simulink model "eVTOL_PX4_2023b"  (R2024b)
settings: Solver=ode4  StartTime=0  StopTime=inf  FixedStep=0.01  RelTol=1e-3
values from neighbouring files (symbols this model uses):
  aDl =     [initdata.mat]
  aDr =     [initdata.mat]
  aDyn =     [initdata.mat]
  Airport = init_airport('PHNL')    [initdata_HIL_eVTOL.m]
  aLat =     [initdata.mat]
  aLon =     [initdata.mat]
  D = Prop.D    [EOM_dt_MC.m]    (also in EOM_get_alf_dt_de_prop_evtol.m = CD * QS)
  dt0 = X(2)    [EOM_get_alf_dt_de_prop_evtol.m]    (also in initdata.mat = 0.258252593971; initdata_HIL_eVTOL.m = EOM_dt_MC)
  EAS0 = TAS0 / EAS2TAS    [initdata_HIL_eVTOL.m]
  FCS = init_FCS    [initdata_HIL_eVTOL.m]
  General = init_layoutdata    [EOM_dt_MC.m]    (also in build_optimized_CA.m; initdata.mat = ; initdata_HIL_eVTOL.m)
  h0 = Con(1)    [EOM_get_alf_dt_de_prop_evtol.m]    (also in initdata.mat = 450; initdata_HIL_eVTOL.m = 50)
  mass = Con(3)    [EOM_get_alf_dt_de_prop_evtol.m]    (also in initdata.mat = 2255.54; initdata_HIL_eVTOL.m = 7)
  Motor = init_motor_evtol    [EOM_dt_MC.m]    (also in initdata.mat = []; initdata_HIL_eVTOL.m)
  Prop = init_propeller_evtol_new    [EOM_dt_MC.m]    (also in initdata_HIL_eVTOL.m)
  R2D = 180/pi    (= 57.2957795131)    [EOM_get_alf_dt_de_prop_evtol.m]    (also in init_FCS.m; init_aerodata_evtol.m; init_airport.m; initdata.mat)
  SAMPLE_TIME = 0.01    [initdata_HIL_eVTOL.m]
  theta0 = -0.0510981441662    [initdata.mat]
undefined symbols (not defined in the file or in its folder): A1, aDa, aDe, aero, asbhl20env, B1, C1, de0, Earth, Environment, INIT_Data, InitData, Kd, Kp, magnitude, Newton, pProp, Raphson, Tc, WGS84
libraries: simulink_extras x63, vrlib x48, sharedtransform x28, simulink x22, slpidlib x20, sharedutil x20, matrix_library x18, aerolibwindfilters x12, aerolibobsolete x8, aerolibasang x8, aerolibatmos2 x6, aerolibfltsims x6
(part 14 of 17)

== system eVTOL_PX4_2023b/Subsystem2/airframe/force moment/aero F&M in body axis/Aerodynamic Coefficients ==
  Incid : Inport
  mach : Inport  Port=2
  pqrn : Inport  Port=3
  alphaDot_n : Inport  Port=4
  Act_surface : Inport  Port=5
  Actuator Increments : Subsystem  AncestorBlock=|
      | asbhl20vehicle/Vehicle/Aerodynamic/Aerodynamic
      | Coefficients/Actuator
      | Increments
      settings: LibrarySourceBlock=|
      | asbhl20vehicle/Vehicle/Aerodynamic/Aerodynamic
      | Coefficients/Actuator
      | Increments
  Basic Coefficients : Subsystem  AncestorBlock=asbhl20vehicle/Vehicle/Aerodynamic/Aerodynamic Coefficients/Datum Coefficients
      settings: LibrarySourceBlock=|
      | asbhl20vehicle/Vehicle/Aerodynamic/Aerodynamic
      | Coefficients/Datum Coefficients
  Body Rate Damping : Subsystem  AncestorBlock=|
      | asbhl20vehicle/Vehicle/Aerodynamic/Aerodynamic
      | Coefficients/Body Rate
      | Damping
      settings: LibrarySourceBlock=|
      | asbhl20vehicle/Vehicle/Aerodynamic/Aerodynamic
      | Coefficients/Body Rate
      | Damping
  CLCDCY-CXCYCZ : Subsystem
  Divide : Product  Inputs=*/
  K : Scope
  Mux1 : Mux  Inputs=2
  Scope{1..5} (5 alike) : Scope
  Selector : Selector  InputPortWidth=6  IndexOptions=Index vector (dialog)  Indices=[1 2 3]  OutputSizes=1
  Selector1 : Selector  InputPortWidth=6  IndexOptions=Index vector (dialog)  Indices=[4 5 6]  OutputSizes=1
  Selector2 : Selector  InputPortWidth=3  IndexOptions=Index vector (dialog)  Indices=1  OutputSizes=1
  Selector3 : Selector  InputPortWidth=3  IndexOptions=Index vector (dialog)  Indices=2  OutputSizes=1
  Sum : Sum  Inputs=3  InputSameDT=on  SaturateOnIntegerOverflow=on  OutDataTypeStr=Inherit: Same as first input
  Coeff : Outport  InitialOutput=0  VectorParamsAs1DForOutWhenUnconnected=off
  wires:
  CLCDCY-CXCYCZ/1(Cl_XYZ) -> Scope1/1, Mux1/1
  Selector1/1 -> Mux1/2, Scope5/1
  Basic Coefficients/1(cl) -> Sum/1, Scope2/1
  Selector2/1 -> Divide/1  "CL"
  Body Rate Damping/1(cl) -> Sum/3, Scope4/1
  alphaDot_n/1 -> Body Rate Damping/3(alphaDot_n)
  Mux1/1 -> Coeff/1
  pqrn/1 -> Body Rate Damping/2(pqrn)
  Actuator Increments/1(cl) -> Sum/2, Scope3/1
  Selector/1 -> Selector3/1, Selector2/1, CLCDCY-CXCYCZ/2(Cl_LDY)
  Selector3/1 -> Divide/2  "CD"
  Sum/1 -> Selector/1, Selector1/1
  Divide/1 -> K/1
  Incid/1 -> Actuator Increments/2(incid), CLCDCY-CXCYCZ/1(Incid), Body Rate Damping/1(Incid), Basic Coefficients/1(Incid)
  Act_surface/1 -> Actuator Increments/1(Actuators)
  mach/1 -> Basic Coefficients/2(mach)

== system eVTOL_PX4_2023b/Subsystem2/airframe/force moment/aero F&M in body axis/nonunit value ==
  V : Inport
  pqr : Inport  Port=2
  alphaDot : Inport  Port=3
  CA : Constant  Value=General.MAC
  Demux2 : Demux  Outputs=3
      settings: DisplayOption=none
  Gain : Gain  Gain=2  SaturateOnIntegerOverflow=on  OutDataTypeStr=Inherit: Same as input  ParamDataTypeStr=Inherit: Same as input
  Mux18 : Mux  Inputs=3
  Product{1..4} (4 alike) : Product  Inputs=/**  SaturateOnIntegerOverflow=on  OutDataTypeStr=Inherit: Same as first input
  b : Constant  Value=General.b
  pqr_n : Outport  VectorParamsAs1DForOutWhenUnconnected=off
  alphaDot_n : Outport  Port=2  VectorParamsAs1DForOutWhenUnconnected=off
  wires:
  pqr/1 -> Demux2/1
  V/1 -> Gain/1
  Product4/1 -> Mux18/2
  Product2/1 -> Mux18/3
  Gain/1 -> Product1/1, Product2/1, Product3/1, Product4/1
  b/1 -> Product1/2, Product2/2
  Demux2/3 -> Product2/3  "r"
  Demux2/2 -> Product4/3  "q"
  Demux2/1 -> Product1/3  "p"
  CA/1 -> Product4/2, Product3/2
  Mux18/1 -> pqr_n/1
  Product1/1 -> Mux18/1
  alphaDot/1 -> Product3/3
  Product3/1 -> alphaDot_n/1

== system eVTOL_PX4_2023b/UAV/airframe/Flight Conditions/Incidence, Sideslip, & Airspeed/Subsystem ==
  V : Inport
  Demux1 : Demux  Outputs=3
      settings: DisplayOption=none
  Terminator : Terminator
  w : Outport  VectorParamsAs1DForOutWhenUnconnected=off
  U : Outport  Port=2  VectorParamsAs1DForOutWhenUnconnected=off
  wires:
  Demux1/3 -> w/1
  Demux1/2 -> Terminator/1
  V/1 -> Demux1/1
  Demux1/1 -> U/1

== system eVTOL_PX4_2023b/UAV/airframe/Flight Conditions/Incidence, Sideslip, & Airspeed/Subsystem1 ==
  V : Inport
  Demux1 : Demux  Outputs=3
      settings: DisplayOption=none
  Terminator : Terminator
  Terminator1 : Terminator
  v : Outport  VectorParamsAs1DForOutWhenUnconnected=off
  wires:
  Demux1/1 -> Terminator/1
  V/1 -> Demux1/1
  Demux1/2 -> v/1
  Demux1/3 -> Terminator1/1

== system eVTOL_PX4_2023b/UAV/airframe/Flight Conditions/Incidence, Sideslip, & Airspeed/dot ==
  Vb : Inport
  Demux1 : Demux  Outputs=3
  Product : Product  RndMeth=Zero
  Product1 : Product  RndMeth=Zero
  Product2 : Product  RndMeth=Zero
  Sum : Sum  Inputs=+++
  dot : Outport  VectorParamsAs1DForOutWhenUnconnected=off
  wires:
  Product2/1 -> Sum/3
  Demux1/3 -> Product2/2, Product2/1
  Product/1 -> Sum/1
  Product1/1 -> Sum/2
  Sum/1 -> dot/1
  Vb/1 -> Demux1/1
  Demux1/1 -> Product/2, Product/1
  Demux1/2 -> Product1/1, Product1/2

== system eVTOL_PX4_2023b/UAV/airframe/force moment/Gear&FM in body axis/F&M  Front Gear Left ==
  PlantData : Inport
  dg : Inport  Port=2
  Bus Selector : BusSelector  OutputSignals=Xe,DCM_be,Vb,pqr,Euler
  Constant1 : Constant  Value=General.CD0_gear_taxi
  Constant{3,5..6,9,11} (5 alike) : Constant  Value=0
  Constant15 : Constant  Value=General.h_runway
  Constant2 : Constant  Value=General.pos_fgl
  Constant4 : Constant  Value=General.Kb
  Constant7 : Constant  Value=General.Kf
  Constant8 : Constant  Value=General.Cf
  Cross Product : vrlib/Utilities/Cross Product
  Cross Product1 : vrlib/Utilities/Cross Product
  Divide : Product  Inputs=*/
  F_fgl scp : Scope
  F_in_earth scp : Scope
  F_in_earth scp1 : Scope
  F_in_gear scp : Scope
  Gain1 : Gain  Gain=-1
  Gain2 : Gain  Gain=-1
  Gain3 : Gain  Gain=-1
  "Lge, e 2 gear" : sharedtransform/Rotation Angles to Direction Cosine Matrix  rotationOrder=XYZ  aMode=aMode
  M_fgr scp : Scope
  Math Function : Math  Operator=transpose  SignedPower=on
  Math Function1 : Math  Operator=transpose  SignedPower=on
  Math Function2 : Math  Operator=transpose  SignedPower=on
  Mux{,1..3} (4 alike) : Mux  Inputs=3
  Product{1,4..6} (4 alike) : Product
  Product{2..3,7..11} (7 alike) : Product  Multiplication=Matrix(*)
  Selector1 : Selector  InputPortWidth=3  IndexOptions=Index vector (dialog)  Indices=2  OutputSizes=1
  Selector2 : Selector  InputPortWidth=3  IndexOptions=Index vector (dialog)  Indices=1  OutputSizes=1
  Selector{3..7} (5 alike) : Selector  InputPortWidth=3  IndexOptions=Index vector (dialog)  Indices=3  OutputSizes=1
  Sum{1..3,5,7} (5 alike) : Sum  Inputs=|++
  Sum4 : Sum  Inputs=|+-
  Sum6 : Sum  Inputs=-+|
  Switch1 : Switch  SaturateOnIntegerOverflow=off  InputSameDT=off
  Trigonometric Function : Trigonometry  Operator=atan
  beta fgl{,1..3} (4 alike) : Scope
  hrel_fgl : Scope
  F_fgl : Outport  VectorParamsAs1DForOutWhenUnconnected=off
  M_fgl : Outport  Port=2  VectorParamsAs1DForOutWhenUnconnected=off
  wires:
  Selector5/1 -> Sum2/2
  Constant3/1 -> Mux/1, Mux/2
  Bus Selector/3 -> Sum7/1  "<Vb>"
  Product3/1 -> beta fgl1/1, Selector2/1, Selector1/1, Gain1/1
  Cross Product/1 -> M_fgl/1, M_fgr scp/1
  Math Function2/1 -> Product7/1, Product9/1
  Product5/1 -> Mux1/2
  dg/1 -> Mux2/3, Sum5/1
  Constant7/1 -> Product4/2
  Sum5/1 -> Mux3/3
  Constant5/1 -> Mux2/2, Mux2/1
  Sum1/1 -> Product8/2
  Constant4/1 -> Product5/1
  Selector4/1 -> Sum3/2
  Sum3/1 -> Switch1/3
  Constant11/1 -> Mux3/2, Mux3/1
  Mux/1 -> Sum1/1
  Mux3/1 -> "Lge, e 2 gear"/1
  Switch1/1 -> Gain2/1, F_in_earth scp1/1, Mux/3  "Fz_fgl"
  Constant1/1 -> Mux1/1
  Product6/1 -> Selector4/1
  Product10/1 -> Product7/2
  Selector3/1 -> Sum5/2
  "Lge, e 2 gear"/1 -> Product3/1, Math Function2/1
  Divide/1 -> Trigonometric Function/1
  Cross Product1/1 -> Sum7/2
  Constant6/1 -> Switch1/1
  Sum2/1 -> beta fgl3/1, Product5/2
  Product9/1 -> Sum1/2, F_in_earth scp/1  "F_in_earth"
  Product4/1 -> Sum3/1
  Selector1/1 -> Divide/1
  Product1/1 -> Product9/2, F_in_gear scp/1  "F_in_gear"
  Gain2/1 -> Product1/1
  Selector2/1 -> Divide/2
  Mux1/1 -> Product1/2  "F_in_gear"
  Gain1/1 -> Product6/2
  Constant9/1 -> Mux1/3
  Sum7/1 -> Product2/2
  Product8/1 -> F_fgl/1, F_fgl scp/1, Cross Product/2  "F_support_in_b"
  Mux2/1 -> Product10/2
  Bus Selector/5 -> Selector3/1  "<Euler>"
  Trigonometric Function/1 -> Sum2/1, beta fgl/1  "beta"
  Constant8/1 -> Product6/1
  Math Function1/1 -> Product2/1
  Product2/1 -> beta fgl2/1, Product3/2
  Bus Selector/4 -> Cross Product1/1  "<pqr>"
  Product7/1 -> Selector5/1
  Sum4/1 -> Product4/1, Switch1/2, hrel_fgl/1  "hrel_fgl"
  Bus Selector/1 -> Selector7/1  "<Xe>"
  Constant15/1 -> Sum6/1
  Selector6/1 -> Sum4/2  "z_cg2fgl_in_e_free"
  Product11/1 -> Selector6/1
  Selector7/1 -> Gain3/1
  Bus Selector/2 -> Product10/1, Product8/1, Math Function1/1, Math Function/1  "<DCM_be>"
  Math Function/1 -> Product11/1
  Gain3/1 -> Sum6/2
  Constant2/1 -> Cross Product/1, Product11/2, Cross Product1/2
  Sum6/1 -> Sum4/1  "hrel_cg"
  PlantData/1 -> Bus Selector/1

== system eVTOL_PX4_2023b/UAV/airframe/force moment/Gear&FM in body axis/F&M  Front Gear Right ==
  PlantData : Inport
  dg : Inport  Port=2
  Bus Selector : BusSelector  OutputSignals=Xe,DCM_be,Vb,pqr,Euler
  Constant1 : Constant  Value=General.CD0_gear_taxi
  Constant{3,5..6,9,11} (5 alike) : Constant  Value=0
  Constant15 : Constant  Value=General.h_runway
  Constant2 : Constant  Value=General.pos_fgr
  Constant4 : Constant  Value=General.Kb
  Constant7 : Constant  Value=General.Kf
  Constant8 : Constant  Value=General.Cf
  Cross Product : vrlib/Utilities/Cross Product
  Cross Product1 : vrlib/Utilities/Cross Product
  Divide : Product  Inputs=*/
  F_fgl scp : Scope
  F_in_earth scp : Scope
  F_in_earth scp1 : Scope
  F_in_gear scp : Scope
  Gain1 : Gain  Gain=-1
  Gain2 : Gain  Gain=-1
  Gain3 : Gain  Gain=-1
  "Lge, e 2 gear" : sharedtransform/Rotation Angles to Direction Cosine Matrix  rotationOrder=XYZ  aMode=aMode
  M_fgr scp : Scope
  Math Function : Math  Operator=transpose  SignedPower=on
  Math Function1 : Math  Operator=transpose  SignedPower=on
  Math Function2 : Math  Operator=transpose  SignedPower=on
  Mux{,1..3} (4 alike) : Mux  Inputs=3
  Product{1,4..6} (4 alike) : Product
  Product{2..3,7..11} (7 alike) : Product  Multiplication=Matrix(*)
  Selector1 : Selector  InputPortWidth=3  IndexOptions=Index vector (dialog)  Indices=2  OutputSizes=1
  Selector2 : Selector  InputPortWidth=3  IndexOptions=Index vector (dialog)  Indices=1  OutputSizes=1
  Selector{3..7} (5 alike) : Selector  InputPortWidth=3  IndexOptions=Index vector (dialog)  Indices=3  OutputSizes=1
  Sum{1..3,5,7} (5 alike) : Sum  Inputs=|++
  Sum4 : Sum  Inputs=|+-
  Sum6 : Sum  Inputs=-+|
  Switch1 : Switch  SaturateOnIntegerOverflow=off  InputSameDT=off
  Trigonometric Function : Trigonometry  Operator=atan
  beta fgl{,1..3} (4 alike) : Scope
  hrel_fgl : Scope
  F_fgl : Outport  VectorParamsAs1DForOutWhenUnconnected=off
  M_fgl : Outport  Port=2  VectorParamsAs1DForOutWhenUnconnected=off
  wires:
  Selector5/1 -> Sum2/2
  Constant3/1 -> Mux/1, Mux/2
  Bus Selector/3 -> Sum7/1  "<Vb>"
  Product3/1 -> beta fgl1/1, Selector2/1, Selector1/1, Gain1/1
  Cross Product/1 -> M_fgl/1, M_fgr scp/1
  Math Function2/1 -> Product7/1, Product9/1
  Product5/1 -> Mux1/2
  dg/1 -> Mux2/3, Sum5/1
  Constant7/1 -> Product4/2
  Sum5/1 -> Mux3/3
  Constant5/1 -> Mux2/2, Mux2/1
  Sum1/1 -> Product8/2
  Constant4/1 -> Product5/1
  Selector4/1 -> Sum3/2
  Sum3/1 -> Switch1/3
  Constant11/1 -> Mux3/2, Mux3/1
  Mux/1 -> Sum1/1
  Mux3/1 -> "Lge, e 2 gear"/1
  Switch1/1 -> Gain2/1, F_in_earth scp1/1, Mux/3  "Fz_fgl"
  Constant1/1 -> Mux1/1
  Product6/1 -> Selector4/1
  Product10/1 -> Product7/2
  Selector3/1 -> Sum5/2
  "Lge, e 2 gear"/1 -> Product3/1, Math Function2/1
  Divide/1 -> Trigonometric Function/1
  Cross Product1/1 -> Sum7/2
  Constant6/1 -> Switch1/1
  Sum2/1 -> beta fgl3/1, Product5/2
  Product9/1 -> Sum1/2, F_in_earth scp/1  "F_in_earth"
  Product4/1 -> Sum3/1
  Selector1/1 -> Divide/1
  Product1/1 -> Product9/2, F_in_gear scp/1  "F_in_gear"
  Gain2/1 -> Product1/1
  Selector2/1 -> Divide/2
  Mux1/1 -> Product1/2  "F_in_gear"
  Gain1/1 -> Product6/2
  Constant9/1 -> Mux1/3
  Sum7/1 -> Product2/2
  Product8/1 -> F_fgl/1, F_fgl scp/1, Cross Product/2  "F_support_in_b"
  Mux2/1 -> Product10/2
  Bus Selector/5 -> Selector3/1  "<Euler>"
  Trigonometric Function/1 -> Sum2/1, beta fgl/1  "beta"
  Constant8/1 -> Product6/1
  Math Function1/1 -> Product2/1
  Product2/1 -> beta fgl2/1, Product3/2
  Bus Selector/4 -> Cross Product1/1  "<pqr>"
  Product7/1 -> Selector5/1
  Sum4/1 -> Product4/1, Switch1/2, hrel_fgl/1  "hrel_fgl"
  Bus Selector/1 -> Selector7/1  "<Xe>"
  Constant15/1 -> Sum6/1
  Selector6/1 -> Sum4/2  "z_cg2fgl_in_e_free"
  Product11/1 -> Selector6/1
  Selector7/1 -> Gain3/1
  Bus Selector/2 -> Product10/1, Product8/1, Math Function1/1, Math Function/1  "<DCM_be>"
  Math Function/1 -> Product11/1
  Gain3/1 -> Sum6/2
  Constant2/1 -> Cross Product/1, Product11/2, Cross Product1/2
  Sum6/1 -> Sum4/1  "hrel_cg"
  PlantData/1 -> Bus Selector/1

== system eVTOL_PX4_2023b/UAV/airframe/force moment/Gear&FM in body axis/F&M  Main Gear Left ==
  PlantData : Inport
  dg : Inport  Port=2
  Bus Selector : BusSelector  OutputSignals=Xe,DCM_be,Vb,pqr,Euler
  Constant1 : Constant  Value=General.CD0_gear_taxi
  Constant{3,5..6,9,11} (5 alike) : Constant  Value=0
  Constant15 : Constant  Value=General.h_runway
  Constant2 : Constant  Value=General.pos_mgl
  Constant4 : Constant  Value=General.Kb
  Constant7 : Constant  Value=General.Kf
  Constant8 : Constant  Value=General.Cf
  Cross Product : vrlib/Utilities/Cross Product
  Cross Product1 : vrlib/Utilities/Cross Product
  Divide : Product  Inputs=*/
  F_fgl scp : Scope
  F_in_earth scp : Scope
  F_in_earth scp1 : Scope
  F_in_gear scp : Scope
  Gain1 : Gain  Gain=-1
  Gain2 : Gain  Gain=-1
  Gain3 : Gain  Gain=-1
  "Lge, e 2 gear" : sharedtransform/Rotation Angles to Direction Cosine Matrix  rotationOrder=XYZ  aMode=aMode
  M_fgr scp : Scope
  Math Function : Math  Operator=transpose  SignedPower=on
  Math Function1 : Math  Operator=transpose  SignedPower=on
  Math Function2 : Math  Operator=transpose  SignedPower=on
  Mux{,1..3} (4 alike) : Mux  Inputs=3
  Product{1,4..6} (4 alike) : Product
  Product{2..3,7..11} (7 alike) : Product  Multiplication=Matrix(*)
  Selector1 : Selector  InputPortWidth=3  IndexOptions=Index vector (dialog)  Indices=2  OutputSizes=1
  Selector2 : Selector  InputPortWidth=3  IndexOptions=Index vector (dialog)  Indices=1  OutputSizes=1
  Selector{3..7} (5 alike) : Selector  InputPortWidth=3  IndexOptions=Index vector (dialog)  Indices=3  OutputSizes=1
  Sum{1..3,5,7} (5 alike) : Sum  Inputs=|++
  Sum4 : Sum  Inputs=|+-
  Sum6 : Sum  Inputs=-+|
  Switch1 : Switch  SaturateOnIntegerOverflow=off  InputSameDT=off
  Trigonometric Function : Trigonometry  Operator=atan
  beta fgl{,1..3} (4 alike) : Scope
  hrel_fgl : Scope
  F_fgl : Outport  VectorParamsAs1DForOutWhenUnconnected=off
  M_fgl : Outport  Port=2  VectorParamsAs1DForOutWhenUnconnected=off
  wires:
  Selector5/1 -> Sum2/2
  Constant3/1 -> Mux/1, Mux/2
  Bus Selector/3 -> Sum7/1  "<Vb>"
  Product3/1 -> beta fgl1/1, Selector2/1, Selector1/1, Gain1/1
  Cross Product/1 -> M_fgl/1, M_fgr scp/1
  Math Function2/1 -> Product7/1, Product9/1
  Product5/1 -> Mux1/2
  dg/1 -> Mux2/3, Sum5/1
  Constant7/1 -> Product4/2
  Sum5/1 -> Mux3/3
  Constant5/1 -> Mux2/2, Mux2/1
  Sum1/1 -> Product8/2
  Constant4/1 -> Product5/1
  Selector4/1 -> Sum3/2
  Sum3/1 -> Switch1/3
  Constant11/1 -> Mux3/2, Mux3/1
  Mux/1 -> Sum1/1
  Mux3/1 -> "Lge, e 2 gear"/1
  Switch1/1 -> Gain2/1, F_in_earth scp1/1, Mux/3  "Fz_fgl"
  Constant1/1 -> Mux1/1
  Product6/1 -> Selector4/1
  Product10/1 -> Product7/2
  Selector3/1 -> Sum5/2
  "Lge, e 2 gear"/1 -> Product3/1, Math Function2/1
  Divide/1 -> Trigonometric Function/1
  Cross Product1/1 -> Sum7/2
  Constant6/1 -> Switch1/1
  Sum2/1 -> beta fgl3/1, Product5/2
  Product9/1 -> Sum1/2, F_in_earth scp/1  "F_in_earth"
  Product4/1 -> Sum3/1
  Selector1/1 -> Divide/1
  Product1/1 -> Product9/2, F_in_gear scp/1  "F_in_gear"
  Gain2/1 -> Product1/1
  Selector2/1 -> Divide/2
  Mux1/1 -> Product1/2  "F_in_gear"
  Gain1/1 -> Product6/2
  Constant9/1 -> Mux1/3
  Sum7/1 -> Product2/2
  Product8/1 -> F_fgl/1, F_fgl scp/1, Cross Product/2  "F_support_in_b"
  Mux2/1 -> Product10/2
  Bus Selector/5 -> Selector3/1  "<Euler>"
  Trigonometric Function/1 -> Sum2/1, beta fgl/1  "beta"
  Constant8/1 -> Product6/1
  Math Function1/1 -> Product2/1
  Product2/1 -> beta fgl2/1, Product3/2
  Bus Selector/4 -> Cross Product1/1  "<pqr>"
  Product7/1 -> Selector5/1
  Sum4/1 -> Product4/1, Switch1/2, hrel_fgl/1  "hrel_fgl"
  Bus Selector/1 -> Selector7/1  "<Xe>"
  Constant15/1 -> Sum6/1
  Selector6/1 -> Sum4/2  "z_cg2fgl_in_e_free"
  Product11/1 -> Selector6/1
  Selector7/1 -> Gain3/1
  Bus Selector/2 -> Product10/1, Product8/1, Math Function1/1, Math Function/1  "<DCM_be>"
  Math Function/1 -> Product11/1
  Gain3/1 -> Sum6/2
  Constant2/1 -> Cross Product/1, Product11/2, Cross Product1/2
  Sum6/1 -> Sum4/1  "hrel_cg"
  PlantData/1 -> Bus Selector/1

== system eVTOL_PX4_2023b/UAV/airframe/force moment/Gear&FM in body axis/F&M  Main Gear Right ==
  PlantData : Inport
  dg : Inport  Port=2
  Bus Selector : BusSelector  OutputSignals=Xe,DCM_be,Vb,pqr,Euler
  Constant1 : Constant  Value=General.CD0_gear_taxi
  Constant{3,5..6,9,11} (5 alike) : Constant  Value=0
  Constant15 : Constant  Value=General.h_runway
  Constant2 : Constant  Value=General.pos_mgr
  Constant4 : Constant  Value=General.Kb
  Constant7 : Constant  Value=General.Kf
  Constant8 : Constant  Value=General.Cf
  Cross Product : vrlib/Utilities/Cross Product
  Cross Product1 : vrlib/Utilities/Cross Product
  Divide : Product  Inputs=*/
  F_fgl scp : Scope
  F_in_earth scp : Scope
  F_in_earth scp1 : Scope
  F_in_gear scp : Scope
  Gain1 : Gain  Gain=-1
  Gain2 : Gain  Gain=-1
  Gain3 : Gain  Gain=-1
  "Lge, e 2 gear" : sharedtransform/Rotation Angles to Direction Cosine Matrix  rotationOrder=XYZ  aMode=aMode
  M_fgr scp : Scope
  Math Function : Math  Operator=transpose  SignedPower=on
  Math Function1 : Math  Operator=transpose  SignedPower=on
  Math Function2 : Math  Operator=transpose  SignedPower=on
  Mux{,1..3} (4 alike) : Mux  Inputs=3
  Product{1,4..6} (4 alike) : Product
  Product{2..3,7..11} (7 alike) : Product  Multiplication=Matrix(*)
  Selector1 : Selector  InputPortWidth=3  IndexOptions=Index vector (dialog)  Indices=2  OutputSizes=1
  Selector2 : Selector  InputPortWidth=3  IndexOptions=Index vector (dialog)  Indices=1  OutputSizes=1
  Selector{3..7} (5 alike) : Selector  InputPortWidth=3  IndexOptions=Index vector (dialog)  Indices=3  OutputSizes=1
  Sum{1..3,5,7} (5 alike) : Sum  Inputs=|++
  Sum4 : Sum  Inputs=|+-
  Sum6 : Sum  Inputs=-+|
  Switch1 : Switch  SaturateOnIntegerOverflow=off  InputSameDT=off
  Trigonometric Function : Trigonometry  Operator=atan
  beta fgl{,1..3} (4 alike) : Scope
  hrel_fgl : Scope
  F_fgl : Outport  VectorParamsAs1DForOutWhenUnconnected=off
  M_fgl : Outport  Port=2  VectorParamsAs1DForOutWhenUnconnected=off
  wires:
  Selector5/1 -> Sum2/2
  Constant3/1 -> Mux/1, Mux/2
  Bus Selector/3 -> Sum7/1  "<Vb>"
  Product3/1 -> beta fgl1/1, Selector2/1, Selector1/1, Gain1/1
  Cross Product/1 -> M_fgl/1, M_fgr scp/1
  Math Function2/1 -> Product7/1, Product9/1
  Product5/1 -> Mux1/2
  dg/1 -> Mux2/3, Sum5/1
  Constant7/1 -> Product4/2
  Sum5/1 -> Mux3/3
  Constant5/1 -> Mux2/2, Mux2/1
  Sum1/1 -> Product8/2
  Constant4/1 -> Product5/1
  Selector4/1 -> Sum3/2
  Sum3/1 -> Switch1/3
  Constant11/1 -> Mux3/2, Mux3/1
  Mux/1 -> Sum1/1
  Mux3/1 -> "Lge, e 2 gear"/1
  Switch1/1 -> Gain2/1, F_in_earth scp1/1, Mux/3  "Fz_fgl"
  Constant1/1 -> Mux1/1
  Product6/1 -> Selector4/1
  Product10/1 -> Product7/2
  Selector3/1 -> Sum5/2
  "Lge, e 2 gear"/1 -> Product3/1, Math Function2/1
  Divide/1 -> Trigonometric Function/1
  Cross Product1/1 -> Sum7/2
  Constant6/1 -> Switch1/1
  Sum2/1 -> beta fgl3/1, Product5/2
  Product9/1 -> Sum1/2, F_in_earth scp/1  "F_in_earth"
  Product4/1 -> Sum3/1
  Selector1/1 -> Divide/1
  Product1/1 -> Product9/2, F_in_gear scp/1  "F_in_gear"
  Gain2/1 -> Product1/1
  Selector2/1 -> Divide/2
  Mux1/1 -> Product1/2  "F_in_gear"
  Gain1/1 -> Product6/2
  Constant9/1 -> Mux1/3
  Sum7/1 -> Product2/2
  Product8/1 -> F_fgl/1, F_fgl scp/1, Cross Product/2  "F_support_in_b"
  Mux2/1 -> Product10/2
  Bus Selector/5 -> Selector3/1  "<Euler>"
  Trigonometric Function/1 -> Sum2/1, beta fgl/1  "beta"
  Constant8/1 -> Product6/1
  Math Function1/1 -> Product2/1
  Product2/1 -> beta fgl2/1, Product3/2
  Bus Selector/4 -> Cross Product1/1  "<pqr>"
  Product7/1 -> Selector5/1
  Sum4/1 -> Product4/1, Switch1/2, hrel_fgl/1  "hrel_fgl"
  Bus Selector/1 -> Selector7/1  "<Xe>"
  Constant15/1 -> Sum6/1
  Selector6/1 -> Sum4/2  "z_cg2fgl_in_e_free"
  Product11/1 -> Selector6/1
  Selector7/1 -> Gain3/1
  Bus Selector/2 -> Product10/1, Product8/1, Math Function1/1, Math Function/1  "<DCM_be>"
  Math Function/1 -> Product11/1
  Gain3/1 -> Sum6/2
  Constant2/1 -> Cross Product/1, Product11/2, Cross Product1/2
  Sum6/1 -> Sum4/1  "hrel_cg"
  PlantData/1 -> Bus Selector/1

== system eVTOL_PX4_2023b/UAV/airframe/force moment/Thrust in body axis1/plr_l ==
  pos : Inport
  Euler : Inport  Port=2
  thrust : Inport  Port=3
  rpm : Inport  Port=4
  3x3 Cross Product : sharedutil/3x3 Cross Product  aMode=aMode
  Constant1 : Constant  Value=0
  Constant4 : Constant  Value=0
  Ix : Gain  Gain=0.5*0.035*0.2032^2
  Mux1 : Mux  Inputs=3
  Mux2 : Mux  Inputs=3
  Product5 : Product  Multiplication=Matrix(*)  RndMeth=Zero
  Rotation Angles to Direction Cosine Matrix : sharedtransform/Rotation Angles to Direction Cosine Matrix  rotationOrder=ZYX  aMode=aMode
  Sum : Sum  Inputs=++|
  pi/30 : Gain  Gain=pi/30
  f : Outport  VectorParamsAs1DForOutWhenUnconnected=off
  m : Outport  Port=2  VectorParamsAs1DForOutWhenUnconnected=off
  wires:
  Mux1/1 -> f/1, Product5/2
  Euler/1 -> Rotation Angles to Direction Cosine Matrix/1
  Constant4/1 -> Mux1/3, Mux1/2
  thrust/1 -> Mux1/1
  Rotation Angles to Direction Cosine Matrix/1 -> Product5/1
  pos/1 -> 3x3 Cross Product/1
  3x3 Cross Product/1 -> Sum/2
  Product5/1 -> 3x3 Cross Product/2
  Sum/1 -> m/1
  rpm/1 -> pi/30/1
  pi/30/1 -> Ix/1  "omega"
  Ix/1 -> Mux2/1
  Constant1/1 -> Mux2/2, Mux2/3
  Mux2/1 -> Sum/1

== system eVTOL_PX4_2023b/UAV/airframe/force moment/Thrust in body axis1/plr_r ==
  pos : Inport
  Euler : Inport  Port=2
  thrust : Inport  Port=3
  rpm : Inport  Port=4
  -1 : Gain  Gain=-1
  3x3 Cross Product : sharedutil/3x3 Cross Product  aMode=aMode
  Constant1 : Constant  Value=0
  Constant4 : Constant  Value=0
  Ix : Gain  Gain=0.5*0.035*0.2032^2
  Mux1 : Mux  Inputs=3
  Mux2 : Mux  Inputs=3
  Product5 : Product  Multiplication=Matrix(*)  RndMeth=Zero
  Rotation Angles to Direction Cosine Matrix : sharedtransform/Rotation Angles to Direction Cosine Matrix  rotationOrder=ZYX  aMode=aMode
  Sum : Sum  Inputs=++|
  pi/30 : Gain  Gain=pi/30
  f : Outport  VectorParamsAs1DForOutWhenUnconnected=off
  m : Outport  Port=2  VectorParamsAs1DForOutWhenUnconnected=off
  wires:
  Product5/1 -> 3x3 Cross Product/2
  3x3 Cross Product/1 -> Sum/2
  pos/1 -> 3x3 Cross Product/1
  Rotation Angles to Direction Cosine Matrix/1 -> Product5/1
  thrust/1 -> Mux1/1
  Constant4/1 -> Mux1/2, Mux1/3
  Euler/1 -> Rotation Angles to Direction Cosine Matrix/1
  Mux1/1 -> Product5/2, f/1
  rpm/1 -> pi/30/1
  pi/30/1 -> Ix/1  "omega"
  Ix/1 -> -1/1
  Constant1/1 -> Mux2/2, Mux2/3
  Sum/1 -> m/1
  Mux2/1 -> Sum/1
  -1/1 -> Mux2/1

== system eVTOL_PX4_2023b/UAV/airframe/force moment/aero F&M in body axis/Aerodynamic Coefficients ==
  Incid : Inport
  pqrn : Inport  Port=2
  alphaDot_n : Inport  Port=3
  Actuators : Inport  Port=4
  Actuator Increments : Subsystem  AncestorBlock=|
      | asbhl20vehicle/Vehicle/Aerodynamic/Aerodynamic
      | Coefficients/Actuator
      | Increments
  Basic Coefficients : Subsystem  AncestorBlock=asbhl20vehicle/Vehicle/Aerodynamic/Aerodynamic Coefficients/Datum Coefficients
  Body Rate Damping : Subsystem  AncestorBlock=|
      | asbhl20vehicle/Vehicle/Aerodynamic/Aerodynamic
      | Coefficients/Body Rate
      | Damping
  Divide : Product  Inputs=*/
  Mux1 : Mux  Inputs=2
  Scope1 : Scope
  Scope2 : Scope
  Selector : Selector  InputPortWidth=6  IndexOptions=Index vector (dialog)  Indices=[1 2 3]  OutputSizes=1
  Selector1 : Selector  InputPortWidth=6  IndexOptions=Index vector (dialog)  Indices=[4 5 6]  OutputSizes=1
  Selector2 : Selector  InputPortWidth=6  IndexOptions=Index vector (dialog)  Indices=1  OutputSizes=1
  Selector3 : Selector  InputPortWidth=6  IndexOptions=Index vector (dialog)  Indices=2  OutputSizes=1
  Sum : Sum  Inputs=3  InputSameDT=on  SaturateOnIntegerOverflow=on  OutDataTypeStr=Inherit: Same as first input
  To Workspace : ToWorkspace  VariableName=L1Dscp  SampleTime=-1
      settings: Decimation=800
  body axis forces ?????????? : Subsystem
  Coeff : Outport  InitialOutput=0  VectorParamsAs1DForOutWhenUnconnected=off
  wires:
  Sum/1 -> Selector2/1, Selector1/1, Selector/1, Selector3/1
  Basic Coefficients/1(cl) -> Scope2/1, Sum/1
  Body Rate Damping/1(cl) -> Sum/3
  Incid/1 -> body axis forces ??????????/1(Incid), Basic Coefficients/1(Incid)
  pqrn/1 -> Body Rate Damping/1(pqrn)
  Actuators/1 -> Actuator Increments/1(Actuators)
  Actuator Increments/1(cl) -> Sum/2
  body axis forces ??????????/1(Cl_XYZ) -> Scope1/1, Mux1/1
  Selector1/1 -> Mux1/2
  Mux1/1 -> Coeff/1
  Selector/1 -> body axis forces ??????????/2(Cl_LDY)
  alphaDot_n/1 -> Body Rate Damping/2(alphaDot_n)
  Selector2/1 -> Divide/1
  Selector3/1 -> Divide/2
  Divide/1 -> To Workspace/1

== system eVTOL_PX4_2023b/UAV/airframe/force moment/aero F&M in body axis/nonunit value ==
  V : Inport
  pqrWind : Inport  Port=2
  alphaDot : Inport  Port=3
  CA : Constant  Value=General.MAC
  Demux2 : Demux  Outputs=3
      settings: DisplayOption=none
  Gain : Gain  Gain=2  SaturateOnIntegerOverflow=on  OutDataTypeStr=Inherit: Same as input  ParamDataTypeStr=Inherit: Same as input
  Mux18 : Mux  Inputs=3
  Product{1..4} (4 alike) : Product  Inputs=/**  SaturateOnIntegerOverflow=on  OutDataTypeStr=Inherit: Same as first input
  b : Constant  Value=General.b
  pqr_n : Outport  VectorParamsAs1DForOutWhenUnconnected=off
  alphaDot_n : Outport  Port=2  VectorParamsAs1DForOutWhenUnconnected=off
  wires:
  pqrWind/1 -> Demux2/1
  V/1 -> Gain/1
  Product4/1 -> Mux18/2
  Product2/1 -> Mux18/3
  Gain/1 -> Product1/1, Product4/1, Product2/1, Product3/1
  b/1 -> Product1/2, Product2/2
  Demux2/3 -> Product2/3
  Demux2/2 -> Product4/3
  Demux2/1 -> Product1/3
  CA/1 -> Product4/2, Product3/2
  Mux18/1 -> pqr_n/1
  Product1/1 -> Mux18/1
  alphaDot/1 -> Product3/3
  Product3/1 -> alphaDot_n/1

== system eVTOL_PX4_2023b/FCS/MC/ADRC theta/TD/fhan/fsg ==
  x : Inport
  d : Inport  Port=2
  Gain2 : Gain  Gain=0.5
  Sign1 : Signum
  Sign2 : Signum
  Sum4 : Sum  Inputs=|++
  Sum5 : Sum  Inputs=|+-
  Sum6 : Sum  Inputs=|+-
  fsg : Outport
  wires:
  d/1 -> Sum4/2, Sum5/2
  Sum6/1 -> Gain2/1
  Sign2/1 -> Sum6/2
  x/1 -> Sum5/1, Sum4/1
  Sum4/1 -> Sign1/1
  Sign1/1 -> Sum6/1
  Gain2/1 -> fsg/1
  Sum5/1 -> Sign2/1

== system eVTOL_PX4_2023b/FCS/MC/ADRC theta/TD/fhan/fsg1 ==
  x : Inport
  d : Inport  Port=2
  Gain2 : Gain  Gain=0.5
  Sign1 : Signum
  Sign2 : Signum
  Sum4 : Sum  Inputs=|++
  Sum5 : Sum  Inputs=|+-
  Sum6 : Sum  Inputs=|+-
  fsg : Outport
  wires:
  Sum5/1 -> Sign2/1
  Gain2/1 -> fsg/1
  Sign1/1 -> Sum6/1
  Sum4/1 -> Sign1/1
  x/1 -> Sum4/1, Sum5/1
  Sign2/1 -> Sum6/2
  Sum6/1 -> Gain2/1
  d/1 -> Sum5/2, Sum4/2

== system eVTOL_PX4_2023b/Subsystem1/Environment/Wind Models/Dryden Wind Turbulence Model (Continuous (+q -r))/RMS turbulence intensities/High Altitude Intensity ==
  h : Inport
  Medium/High Altitude Intensity : Interpolation_n-D  Table=sigma_vec'  ExtrapMethod=Clip  ValidIndexMayReachLast=on  OutDataTypeStr=double
  PreLook-Up Index Search (altitude) : PreLookup  BreakpointsData=h_vec  BeginIndexSearchUsingPreviousIndexResult=on  UseLastBreakpoint=on  FractionDataTypeStr=double
  PreLook-Up Index Search (prob of exceed) : PreLookup  BreakpointsData=[1:7]  BeginIndexSearchUsingPreviousIndexResult=on  UseLastBreakpoint=on  FractionDataTypeStr=double
  Probability of Exceedance : Constant  Value=TurbProb
  sigma_ug sigma_vg sigma_wg : Outport  InitialOutput=0  VectorParamsAs1DForOutWhenUnconnected=off
  wires:
  PreLook-Up Index Search (prob of exceed)/2 -> Medium/High Altitude Intensity/4
  PreLook-Up Index Search (prob of exceed)/1 -> Medium/High Altitude Intensity/3
  PreLook-Up Index Search (altitude)/2 -> Medium/High Altitude Intensity/2
  PreLook-Up Index Search (altitude)/1 -> Medium/High Altitude Intensity/1
  h/1 -> PreLook-Up Index Search (altitude)/1
  Medium/High Altitude Intensity/1 -> sigma_ug sigma_vg sigma_wg/1
  Probability of Exceedance/1 -> PreLook-Up Index Search (prob of exceed)/1

== system eVTOL_PX4_2023b/Subsystem1/Environment/Wind Models/Dryden Wind Turbulence Model (Continuous (+q -r))/RMS turbulence intensities/Low Altitude Intensity ==
  Windspeed at 20ft (6m) : Inport
  h : Inport  Port=2
  Limit Height h<1000ft : Saturate  UpperLimit=max_height_low  LowerLimit=0
  Low Altitude Intensity : Fcn  Expr=1/(0.177+0.000823*u(1))^0.4
  "sigma_ug, sigma_vg" : Product  InputSameDT=on  SaturateOnIntegerOverflow=on  OutDataTypeStr=Inherit: Same as first input
  "sigma_wg " : Gain  Gain=0.1  SaturateOnIntegerOverflow=on  OutDataTypeStr=Inherit: Same as input  ParamDataTypeStr=Inherit: Same as input
  sigma_ug sigma_vg : Outport  InitialOutput=0  VectorParamsAs1DForOutWhenUnconnected=off
  sigma_wg : Outport  Port=2  InitialOutput=0  VectorParamsAs1DForOutWhenUnconnected=off
  wires:
  "sigma_ug, sigma_vg"/1 -> sigma_ug sigma_vg/1
  h/1 -> Limit Height h<1000ft/1
  Low Altitude Intensity/1 -> "sigma_ug, sigma_vg"/1
  "sigma_wg "/1 -> sigma_wg/1, "sigma_ug, sigma_vg"/2
  Windspeed at 20ft (6m)/1 -> "sigma_wg "/1
  Limit Height h<1000ft/1 -> Low Altitude Intensity/1

== system eVTOL_PX4_2023b/Subsystem1/Environment/Wind Models/Dryden Wind Turbulence Model (Continuous (+q -r))/Select angular rates/Interpolate rates ==
  pgw_h&l : Inport
  qgw_h&l : Inport  Port=2
  rgw_h&l : Inport  Port=3
  DCM : Inport  Port=4
  Wind direction : Inport  Port=5
  Altitude : Inport  Port=6
  Action Port : ActionPort  PropagateVarSize=During execution  ActionPortLabel=else
  Mux : Mux  Inputs=3
  Mux1 : Mux  Inputs=3
  Product1 : Product  Inputs=**/  SaturateOnIntegerOverflow=on  OutDataTypeStr=Inherit: Same as first input
  Selector : Selector  InputPortWidth=2  IndexOptions=Index vector (dialog)  Indices=1  OutputSizes=1
  Selector1 : Selector  InputPortWidth=2  IndexOptions=Index vector (dialog)  Indices=1  OutputSizes=1
  Selector2 : Selector  InputPortWidth=2  IndexOptions=Index vector (dialog)  Indices=1  OutputSizes=1
  Selector3 : Selector  InputPortWidth=2  IndexOptions=Index vector (dialog)  Indices=2  OutputSizes=1
  Selector4 : Selector  InputPortWidth=2  IndexOptions=Index vector (dialog)  Indices=2  OutputSizes=1
  Selector5 : Selector  InputPortWidth=2  IndexOptions=Index vector (dialog)  Indices=2  OutputSizes=1
  Sum : Sum  Inputs=|-+  SaturateOnIntegerOverflow=on
  Sum1 : Sum  Inputs=|+-  SaturateOnIntegerOverflow=on
  Sum2 : Sum  Inputs=-+|  SaturateOnIntegerOverflow=on
  Sum3 : Sum  Inputs=++|  SaturateOnIntegerOverflow=on
  max_height_low : Constant  Value=max_height_low
  min_height_high : Constant  Value=min_height_high
  wind to body transformation : Subsystem
  pgw,qgw,rgw : Outport  InitialOutput=0  VectorParamsAs1DForOutWhenUnconnected=off
  wires:
  Mux/1 -> wind to body transformation/3(pg_l,qg_l,rg_l)
  DCM/1 -> wind to body transformation/1(DCM)
  wind to body transformation/1(pg,qg,rg) -> Sum3/1, Sum2/1
  Sum3/1 -> pgw,qgw,rgw/1
  Product1/1 -> Sum3/2
  Mux1/1 -> Sum2/2
  Sum2/1 -> Product1/1
  Sum1/1 -> Product1/2
  Sum/1 -> Product1/3
  Altitude/1 -> Sum1/1
  min_height_high/1 -> Sum/2
  max_height_low/1 -> Sum1/2, Sum/1
  Wind direction/1 -> wind to body transformation/2(Wind direction)
  Selector3/1 -> Mux1/1
  Selector4/1 -> Mux1/2
  Selector5/1 -> Mux1/3
  pgw_h&l/1 -> Selector/1, Selector3/1
  qgw_h&l/1 -> Selector4/1, Selector1/1
  rgw_h&l/1 -> Selector5/1, Selector2/1
  Selector/1 -> Mux/1
  Selector1/1 -> Mux/2
  Selector2/1 -> Mux/3

== system eVTOL_PX4_2023b/Subsystem1/Environment/Wind Models/Dryden Wind Turbulence Model (Continuous (+q -r))/Select angular rates/Low altitude rates ==
  DCM : Inport
  pgw_h&l : Inport  Port=2
  qgw_h&l : Inport  Port=3
  rgw_h&l : Inport  Port=4
  Wind direction : Inport  Port=5
  Action Port : ActionPort  PropagateVarSize=During execution  ActionPortLabel=if(u1<=max_height_low)
  Mux : Mux  Inputs=3
  Selector : Selector  InputPortWidth=2  IndexOptions=Index vector (dialog)  Indices=1  OutputSizes=1
  Selector1 : Selector  InputPortWidth=2  IndexOptions=Index vector (dialog)  Indices=1  OutputSizes=1
  Selector2 : Selector  InputPortWidth=2  IndexOptions=Index vector (dialog)  Indices=1  OutputSizes=1
  wind to body transformation : Subsystem
  pgw,qgw,rgw : Outport  InitialOutput=0  VectorParamsAs1DForOutWhenUnconnected=off
  wires:
  DCM/1 -> wind to body transformation/1(DCM)
  pgw_h&l/1 -> Selector/1
  qgw_h&l/1 -> Selector1/1
  rgw_h&l/1 -> Selector2/1
  Selector/1 -> Mux/1
  Selector1/1 -> Mux/2
  Selector2/1 -> Mux/3
  Mux/1 -> wind to body transformation/3(pg_l,qg_l,rg_l)
  wind to body transformation/1(pg,qg,rg) -> pgw,qgw,rgw/1
  Wind direction/1 -> wind to body transformation/2(Wind direction)

== system eVTOL_PX4_2023b/Subsystem1/Environment/Wind Models/Dryden Wind Turbulence Model (Continuous (+q -r))/Select angular rates/Medium//High altitude rates ==
  pgw_h&l : Inport
  qgw_h&l : Inport  Port=2
  rgw_h&l : Inport  Port=3
  Action Port : ActionPort  PropagateVarSize=During execution  ActionPortLabel=elseif(u1>=min_height_high)
  Gain : Gain  SaturateOnIntegerOverflow=on  OutDataTypeStr=Inherit: Same as input  ParamDataTypeStr=Inherit: Same as input
  Mux : Mux  Inputs=3
  Selector3 : Selector  InputPortWidth=6  IndexOptions=Index vector (dialog)  Indices=[ 2 4 6]  OutputSizes=1
  pgw,qgw,rgw : Outport  InitialOutput=0  VectorParamsAs1DForOutWhenUnconnected=off
  wires:
  Gain/1 -> pgw,qgw,rgw/1
  Selector3/1 -> Gain/1
  pgw_h&l/1 -> Mux/1
  qgw_h&l/1 -> Mux/2
  rgw_h&l/1 -> Mux/3
  Mux/1 -> Selector3/1

== system eVTOL_PX4_2023b/Subsystem1/Environment/Wind Models/Dryden Wind Turbulence Model (Continuous (+q -r))/Select angular rates/Merge Subsystems ==
  low : Inport
  high : Inport  Port=2
  interpolated : Inport  Port=3
  Demux : Demux  Outputs=3
      settings: DisplayOption=none
  Merge : Merge  Inputs=3
  pgw : Outport  VectorParamsAs1DForOutWhenUnconnected=off
  qgw : Outport  Port=2  VectorParamsAs1DForOutWhenUnconnected=off
  rgw : Outport  Port=3  VectorParamsAs1DForOutWhenUnconnected=off
  wires:
  low/1 -> Merge/1
  high/1 -> Merge/2
  interpolated/1 -> Merge/3
  Demux/2 -> qgw/1
  Demux/3 -> rgw/1
  Demux/1 -> pgw/1
  Merge/1 -> Demux/1

== system eVTOL_PX4_2023b/Subsystem1/Environment/Wind Models/Dryden Wind Turbulence Model (Continuous (+q -r))/Select velocities/Interpolate velocities ==
  ugw_h&l : Inport
  vgw_h&l : Inport  Port=2
  wgw_h&l : Inport  Port=3
  DCM : Inport  Port=4
  Wind direction : Inport  Port=5
  Altitude : Inport  Port=6
  Action Port : ActionPort  PropagateVarSize=During execution  ActionPortLabel=else
  Mux : Mux  Inputs=3
  Mux1 : Mux  Inputs=3
  Product1 : Product  Inputs=**/  SaturateOnIntegerOverflow=on  OutDataTypeStr=Inherit: Same as first input
  Selector : Selector  InputPortWidth=2  IndexOptions=Index vector (dialog)  Indices=1  OutputSizes=1
  Selector1 : Selector  InputPortWidth=2  IndexOptions=Index vector (dialog)  Indices=1  OutputSizes=1
  Selector2 : Selector  InputPortWidth=2  IndexOptions=Index vector (dialog)  Indices=1  OutputSizes=1
  Selector3 : Selector  InputPortWidth=2  IndexOptions=Index vector (dialog)  Indices=2  OutputSizes=1
  Selector4 : Selector  InputPortWidth=2  IndexOptions=Index vector (dialog)  Indices=2  OutputSizes=1
  Selector5 : Selector  InputPortWidth=2  IndexOptions=Index vector (dialog)  Indices=2  OutputSizes=1
  Sum : Sum  Inputs=|-+  SaturateOnIntegerOverflow=on
  Sum1 : Sum  Inputs=|+-  SaturateOnIntegerOverflow=on
  Sum2 : Sum  Inputs=-+|  SaturateOnIntegerOverflow=on
  Sum3 : Sum  Inputs=++|  SaturateOnIntegerOverflow=on
  max_height_low : Constant  Value=max_height_low
  min_height_high : Constant  Value=min_height_high
  wind to body transformation : Subsystem
  ugw,vgw,wgw : Outport  InitialOutput=0  VectorParamsAs1DForOutWhenUnconnected=off
  wires:
  Mux/1 -> wind to body transformation/3(ug_l,vg_l,wg_l)
  Wind direction/1 -> wind to body transformation/2(Wind direction)
  DCM/1 -> wind to body transformation/1(DCM)
  wind to body transformation/1(ug,vg,wg) -> Sum3/1, Sum2/1
  Sum3/1 -> ugw,vgw,wgw/1
  Product1/1 -> Sum3/2
  Mux1/1 -> Sum2/2
  Sum2/1 -> Product1/1
  Sum1/1 -> Product1/2
  Sum/1 -> Product1/3
  Altitude/1 -> Sum1/1
  min_height_high/1 -> Sum/2
  max_height_low/1 -> Sum1/2, Sum/1
  Selector3/1 -> Mux1/1
  Selector4/1 -> Mux1/2
  Selector5/1 -> Mux1/3
  ugw_h&l/1 -> Selector/1, Selector3/1
  vgw_h&l/1 -> Selector4/1, Selector1/1
  wgw_h&l/1 -> Selector5/1, Selector2/1
  Selector/1 -> Mux/1
  Selector1/1 -> Mux/2
  Selector2/1 -> Mux/3

== system eVTOL_PX4_2023b/Subsystem1/Environment/Wind Models/Dryden Wind Turbulence Model (Continuous (+q -r))/Select velocities/Low altitude velocities ==
  DCM : Inport
  ugw_h&l : Inport  Port=2
  vgw_h&l : Inport  Port=3
  wgw_h&l : Inport  Port=4
  Wind direction : Inport  Port=5
  Action Port : ActionPort  PropagateVarSize=During execution  ActionPortLabel=if(u1<=max_height_low)
  Mux : Mux  Inputs=3
  Selector : Selector  InputPortWidth=2  IndexOptions=Index vector (dialog)  Indices=1  OutputSizes=1
  Selector1 : Selector  InputPortWidth=2  IndexOptions=Index vector (dialog)  Indices=1  OutputSizes=1
  Selector2 : Selector  InputPortWidth=2  IndexOptions=Index vector (dialog)  Indices=1  OutputSizes=1
  wind to body transformation : Subsystem
  ugw,vgw,wgw : Outport  InitialOutput=0  VectorParamsAs1DForOutWhenUnconnected=off
  wires:
  Mux/1 -> wind to body transformation/3(ug_l,vg_l,wg_l)
  Selector2/1 -> Mux/3
  wind to body transformation/1(ug,vg,wg) -> ugw,vgw,wgw/1
  Wind direction/1 -> wind to body transformation/2(Wind direction)
  DCM/1 -> wind to body transformation/1(DCM)
  Selector1/1 -> Mux/2
  Selector/1 -> Mux/1
  wgw_h&l/1 -> Selector2/1
  vgw_h&l/1 -> Selector1/1
  ugw_h&l/1 -> Selector/1

== system eVTOL_PX4_2023b/Subsystem1/Environment/Wind Models/Dryden Wind Turbulence Model (Continuous (+q -r))/Select velocities/Medium//High altitude velocities ==
  ugw_h&l : Inport
  vgw_h&l : Inport  Port=2
  wgw_h&l : Inport  Port=3
  Action Port : ActionPort  PropagateVarSize=During execution  ActionPortLabel=elseif(u1>=min_height_high)
  Gain : Gain  SaturateOnIntegerOverflow=on  OutDataTypeStr=Inherit: Same as input  ParamDataTypeStr=Inherit: Same as input
  Mux : Mux  Inputs=3
  Selector3 : Selector  InputPortWidth=6  IndexOptions=Index vector (dialog)  Indices=[ 2 4 6]  OutputSizes=1
  ugw,vgw,wgw : Outport  InitialOutput=0  VectorParamsAs1DForOutWhenUnconnected=off
  wires:
  vgw_h&l/1 -> Mux/2
  Gain/1 -> ugw,vgw,wgw/1
  Selector3/1 -> Gain/1
  Mux/1 -> Selector3/1
  wgw_h&l/1 -> Mux/3
  ugw_h&l/1 -> Mux/1

== system eVTOL_PX4_2023b/Subsystem1/Environment/Wind Models/Dryden Wind Turbulence Model (Continuous (+q -r))/Select velocities/Merge Subsystems ==
  low : Inport
  high : Inport  Port=2
  interpolated : Inport  Port=3
  Demux : Demux  Outputs=3
      settings: DisplayOption=none
  Merge : Merge  Inputs=3
  ugw : Outport  VectorParamsAs1DForOutWhenUnconnected=off
  vgw : Outport  Port=2  VectorParamsAs1DForOutWhenUnconnected=off
  wgw : Outport  Port=3  VectorParamsAs1DForOutWhenUnconnected=off
  wires:
  Merge/1 -> Demux/1
  Demux/1 -> ugw/1
  Demux/3 -> wgw/1
  Demux/2 -> vgw/1
  interpolated/1 -> Merge/3
  high/1 -> Merge/2
  low/1 -> Merge/1

== system eVTOL_PX4_2023b/Subsystem1/Environment/Wind Models/Dryden Wind Turbulence Model (Continuous (+q -r))/Turbulence scale lengths/Low altitude scale length ==
  h : Inport
  Limit Function 10ft to 1000ft : Saturate  UpperLimit=max_height_low  LowerLimit=10
  Low Altitude Scale Length : Fcn  Expr=u(1)/(0.177+0.000823*u(1))^1.2
  L_ug L_vg : Outport  InitialOutput=0  VectorParamsAs1DForOutWhenUnconnected=off
  L_wg : Outport  Port=2  InitialOutput=0  VectorParamsAs1DForOutWhenUnconnected=off
  wires:
  h/1 -> Limit Function 10ft to 1000ft/1
  Low Altitude Scale Length/1 -> L_ug L_vg/1
  Limit Function 10ft to 1000ft/1 -> L_wg/1, Low Altitude Scale Length/1

== system eVTOL_PX4_2023b/Subsystem1/Environment/Wind Models/Dryden Wind Turbulence Model (Continuous (+q -r))/Turbulence scale lengths/Medium//High altitude scale length ==
  Length Conversion : Subsystem
  Medium/High Altitude : Constant  Value=L_high
  L_ug L_vg L_wg : Outport  Unit=ft  InitialOutput=0  VectorParamsAs1DForOutWhenUnconnected=off
  wires:
  Medium/High Altitude/1 -> Length Conversion/1(in)
  Length Conversion/1(out) -> L_ug L_vg L_wg/1

== system eVTOL_PX4_2023b/Subsystem1/Environment1/Wind Models/Dryden Wind Turbulence Model (Continuous (+q -r))/RMS turbulence intensities/High Altitude Intensity ==
  h : Inport
  Medium/High Altitude Intensity : Interpolation_n-D  Table=sigma_vec'  ExtrapMethod=Clip  ValidIndexMayReachLast=on  OutDataTypeStr=double
  PreLook-Up Index Search (altitude) : PreLookup  BreakpointsData=h_vec  BeginIndexSearchUsingPreviousIndexResult=on  UseLastBreakpoint=on  FractionDataTypeStr=double
  PreLook-Up Index Search (prob of exceed) : PreLookup  BreakpointsData=[1:7]  BeginIndexSearchUsingPreviousIndexResult=on  UseLastBreakpoint=on  FractionDataTypeStr=double
  Probability of Exceedance : Constant  Value=TurbProb
  sigma_ug sigma_vg sigma_wg : Outport  InitialOutput=0  VectorParamsAs1DForOutWhenUnconnected=off
  wires:
  PreLook-Up Index Search (prob of exceed)/2 -> Medium/High Altitude Intensity/4
  PreLook-Up Index Search (prob of exceed)/1 -> Medium/High Altitude Intensity/3
  PreLook-Up Index Search (altitude)/2 -> Medium/High Altitude Intensity/2
  PreLook-Up Index Search (altitude)/1 -> Medium/High Altitude Intensity/1
  h/1 -> PreLook-Up Index Search (altitude)/1
  Medium/High Altitude Intensity/1 -> sigma_ug sigma_vg sigma_wg/1
  Probability of Exceedance/1 -> PreLook-Up Index Search (prob of exceed)/1

== system eVTOL_PX4_2023b/Subsystem1/Environment1/Wind Models/Dryden Wind Turbulence Model (Continuous (+q -r))/RMS turbulence intensities/Low Altitude Intensity ==
  Windspeed at 20ft (6m) : Inport
  h : Inport  Port=2
  Limit Height h<1000ft : Saturate  UpperLimit=max_height_low  LowerLimit=0
  Low Altitude Intensity : Fcn  Expr=1/(0.177+0.000823*u(1))^0.4
  "sigma_ug, sigma_vg" : Product  InputSameDT=on  SaturateOnIntegerOverflow=on  OutDataTypeStr=Inherit: Same as first input
  "sigma_wg " : Gain  Gain=0.1  SaturateOnIntegerOverflow=on  OutDataTypeStr=Inherit: Same as input  ParamDataTypeStr=Inherit: Same as input
  sigma_ug sigma_vg : Outport  InitialOutput=0  VectorParamsAs1DForOutWhenUnconnected=off
  sigma_wg : Outport  Port=2  InitialOutput=0  VectorParamsAs1DForOutWhenUnconnected=off
  wires:
  "sigma_ug, sigma_vg"/1 -> sigma_ug sigma_vg/1
  h/1 -> Limit Height h<1000ft/1
  Low Altitude Intensity/1 -> "sigma_ug, sigma_vg"/1
  "sigma_wg "/1 -> sigma_wg/1, "sigma_ug, sigma_vg"/2
  Windspeed at 20ft (6m)/1 -> "sigma_wg "/1
  Limit Height h<1000ft/1 -> Low Altitude Intensity/1

== system eVTOL_PX4_2023b/Subsystem1/Environment1/Wind Models/Dryden Wind Turbulence Model (Continuous (+q -r))/Select angular rates/Interpolate rates ==
  pgw_h&l : Inport
  qgw_h&l : Inport  Port=2
  rgw_h&l : Inport  Port=3
  DCM : Inport  Port=4
  Wind direction : Inport  Port=5
  Altitude : Inport  Port=6
  Action Port : ActionPort  PropagateVarSize=During execution  ActionPortLabel=else
  Mux : Mux  Inputs=3
  Mux1 : Mux  Inputs=3
  Product1 : Product  Inputs=**/  SaturateOnIntegerOverflow=on  OutDataTypeStr=Inherit: Same as first input
  Selector : Selector  InputPortWidth=2  IndexOptions=Index vector (dialog)  Indices=1  OutputSizes=1
  Selector1 : Selector  InputPortWidth=2  IndexOptions=Index vector (dialog)  Indices=1  OutputSizes=1
  Selector2 : Selector  InputPortWidth=2  IndexOptions=Index vector (dialog)  Indices=1  OutputSizes=1
  Selector3 : Selector  InputPortWidth=2  IndexOptions=Index vector (dialog)  Indices=2  OutputSizes=1
  Selector4 : Selector  InputPortWidth=2  IndexOptions=Index vector (dialog)  Indices=2  OutputSizes=1
  Selector5 : Selector  InputPortWidth=2  IndexOptions=Index vector (dialog)  Indices=2  OutputSizes=1
  Sum : Sum  Inputs=|-+  SaturateOnIntegerOverflow=on
  Sum1 : Sum  Inputs=|+-  SaturateOnIntegerOverflow=on
  Sum2 : Sum  Inputs=-+|  SaturateOnIntegerOverflow=on
  Sum3 : Sum  Inputs=++|  SaturateOnIntegerOverflow=on
  max_height_low : Constant  Value=max_height_low
  min_height_high : Constant  Value=min_height_high
  wind to body transformation : Subsystem
  pgw,qgw,rgw : Outport  InitialOutput=0  VectorParamsAs1DForOutWhenUnconnected=off
  wires:
  Mux/1 -> wind to body transformation/3(pg_l,qg_l,rg_l)
  DCM/1 -> wind to body transformation/1(DCM)
  wind to body transformation/1(pg,qg,rg) -> Sum3/1, Sum2/1
  Sum3/1 -> pgw,qgw,rgw/1
  Product1/1 -> Sum3/2
  Mux1/1 -> Sum2/2
  Sum2/1 -> Product1/1
  Sum1/1 -> Product1/2
  Sum/1 -> Product1/3
  Altitude/1 -> Sum1/1
  min_height_high/1 -> Sum/2
  max_height_low/1 -> Sum1/2, Sum/1
  Wind direction/1 -> wind to body transformation/2(Wind direction)
  Selector3/1 -> Mux1/1
  Selector4/1 -> Mux1/2
  Selector5/1 -> Mux1/3
  pgw_h&l/1 -> Selector/1, Selector3/1
  qgw_h&l/1 -> Selector4/1, Selector1/1
  rgw_h&l/1 -> Selector5/1, Selector2/1
  Selector/1 -> Mux/1
  Selector1/1 -> Mux/2
  Selector2/1 -> Mux/3

== system eVTOL_PX4_2023b/Subsystem1/Environment1/Wind Models/Dryden Wind Turbulence Model (Continuous (+q -r))/Select angular rates/Low altitude rates ==
  DCM : Inport
  pgw_h&l : Inport  Port=2
  qgw_h&l : Inport  Port=3
  rgw_h&l : Inport  Port=4
  Wind direction : Inport  Port=5
  Action Port : ActionPort  PropagateVarSize=During execution  ActionPortLabel=if(u1<=max_height_low)
  Mux : Mux  Inputs=3
  Selector : Selector  InputPortWidth=2  IndexOptions=Index vector (dialog)  Indices=1  OutputSizes=1
  Selector1 : Selector  InputPortWidth=2  IndexOptions=Index vector (dialog)  Indices=1  OutputSizes=1
  Selector2 : Selector  InputPortWidth=2  IndexOptions=Index vector (dialog)  Indices=1  OutputSizes=1
  wind to body transformation : Subsystem
  pgw,qgw,rgw : Outport  InitialOutput=0  VectorParamsAs1DForOutWhenUnconnected=off
  wires:
  DCM/1 -> wind to body transformation/1(DCM)
  pgw_h&l/1 -> Selector/1
  qgw_h&l/1 -> Selector1/1
  rgw_h&l/1 -> Selector2/1
  Selector/1 -> Mux/1
  Selector1/1 -> Mux/2
  Selector2/1 -> Mux/3
  Mux/1 -> wind to body transformation/3(pg_l,qg_l,rg_l)
  wind to body transformation/1(pg,qg,rg) -> pgw,qgw,rgw/1
  Wind direction/1 -> wind to body transformation/2(Wind direction)
